simulink model "model"  (R2015a)
settings: Solver=ode45  StartTime=0.0  StopTime=200  MaxStep=0.1  RelTol=1e-3
values from neighbouring files (symbols this model uses):
  g = 9.81    [balancin.m]
  Id = (1/2)*md*(Re^2+Ri^2)    (= 0.000284581170525)    [balancin.m]
  l = 0.12    [balancin.m]
  ms = 1.1*md    (= 0.102635831993)    [balancin.m]
  R = 0.1    [balancin.m]
settings Model: Creator=Richa  LastModifiedBy=Richa

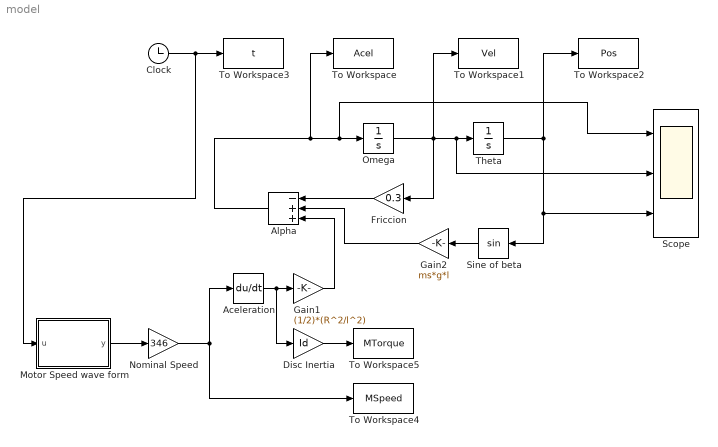
== system model ==
  Aceleration : Derivative
  Alpha : Sum  Inputs=-++
  Clock : Clock
  Disc Inertia : Gain  Gain=Id
  Friccion : Gain  Gain=0.3
  Gain1 : Gain  Gain=(1/2)*(R^2/l^2)
  Gain2 : Gain  Gain=ms*g*l
  Motor Speed wave form : MATLAB Function  TreatAsAtomicUnit=on
  Nominal Speed : Gain  Gain=346
  Omega : Integrator
  Scope : Scope  NumInputPorts=3
      settings: TickLabels=on  ShowLegends=on  YMin=-5~-5~-5  YMax=5~5~5  ScrollMode=on
  Sine of beta : Trigonometry
  Theta : Integrator  InitialCondition=pi/2  LimitOutput=on  UpperSaturationLimit=pi/2  LowerSaturationLimit=-pi/2
  To Workspace : ToWorkspace  VariableName=Acel  SampleTime=-1
  To Workspace1 : ToWorkspace  VariableName=Vel  SampleTime=-1
  To Workspace2 : ToWorkspace  VariableName=Pos  SampleTime=-1
  To Workspace3 : ToWorkspace  VariableName=t  SampleTime=-1
  To Workspace4 : ToWorkspace  VariableName=MSpeed  SampleTime=-1
  To Workspace5 : ToWorkspace  VariableName=MTorque  SampleTime=-1
  wires:
  Omega/1 -> To Workspace1/1, Scope/2, Theta/1, Friccion/1
  Sine of beta/1 -> Gain2/1
  Alpha/1 -> To Workspace/1, Scope/1, Omega/1
  Clock/1 -> Motor Speed wave form/1(u), To Workspace3/1
  Gain1/1 -> Alpha/3
  Gain2/1 -> Alpha/2
  Friccion/1 -> Alpha/1
  Theta/1 -> Sine of beta/1, Scope/3, To Workspace2/1
  Aceleration/1 -> Disc Inertia/1, Gain1/1
  Disc Inertia/1 -> To Workspace5/1
  Motor Speed wave form/1(y) -> Nominal Speed/1
  Nominal Speed/1 -> Aceleration/1, To Workspace4/1

== matlab function model/Motor Speed wave form ==
  data: u input; y output
function y = fcn(u)
y = (1./(1+exp(-u*0.2+5))-(1./(1+exp(-u*3+200))));
